simulink model "balan_model"  (R2018b)
settings: Solver=VariableStepAuto  StartTime=0.0  StopTime=15  FixedStep=0.001  MaxStep=0.01  RelTol=1e-6
undefined symbols (not defined in the file or in its folder): b, cart_d0, cart_d1, cart_d2, cart_d3, cart_d4, cart_n0, cart_n1, cart_n2, d_P_cart_den, d_P_cart_num, d_P_pend_den, d_P_pend_num, DiscIntNeverNeededParam, g, J, k, l, m, M, pend_d0, pend_d1, pend_d2, pend_d3, pend_n0, pend_n1
libraries: simulink_extras x4, simulink x3
settings Model: Creator=Ikarus  LastModifiedBy=Ikarus

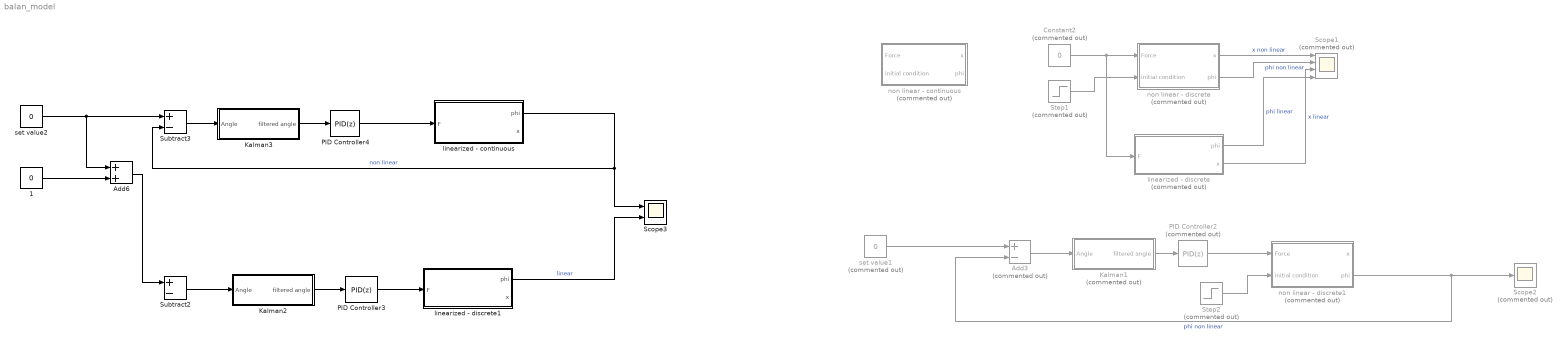
== system balan_model ==
  " 1" : Constant  Value=0  SampleTime=-1
  Add3 : Sum  Commented=on  Inputs=+-
  Add6 : Sum
  Constant2 : Constant  Commented=on  Value=0
  Kalman1 : Subsystem  Commented=on  mask{step_time=0.01}
      mask prompts: step_time "step time"
  Kalman2 : Subsystem  mask{step_time=0.01}
      mask prompts: step_time "step time"
  Kalman3 : Subsystem  mask{step_time=0.01}
      mask prompts: step_time "step time"
  PID Controller2 : simulink/Continuous/PID Controller  Commented=on  Controller=PID  Form=Parallel  TimeDomain=Discrete-time  SampleTime=-1  IntegratorMethod=Forward Euler  FilterMethod=Forward Euler  ControllerParametersSource=internal  P=1235  I=9215  D=40  UseFilter=on  N=868  TunerSelectOption=Transfer Function Based (PID Tuner App)  InitialConditionSource=internal  InitialConditionForIntegrator=0  InitialConditionForFilter=0  DifferentiatorICPrevScaledInput=0  ExternalReset=none  TrackingMode=off  Kt=1  LimitOutput=off  UpperSaturationLimit=inf  LowerSaturationLimit=-inf  LinearizeAsGain=on  AntiWindupMode=none  Kb=1  POutMin=[]  POutMax=[]  IOutMin=[]  IOutMax=[]  DOutMin=[]  DOutMax=[]  NOutMin=[]  NOutMax=[]  SumOutMin=[]  SumOutMax=[]  SaturationOutMin=[]  SaturationOutMax=[]  PParamMin=[]  PParamMax=[]  IParamMin=[]  IParamMax=[]  DParamMin=[]  DParamMax=[]  NParamMin=[]  NParamMax=[]  KbParamMin=[]  KbParamMax=[]  KtParamMin=[]  KtParamMax=[]  KbOutMin=[]  KbOutMax=[]  KtOutMin=[]  KtOutMax=[]  IntegratorOutMin=[]  IntegratorOutMax=[]  FilterOutMin=[]  FilterOutMax=[]  SumI1OutMin=[]  SumI1OutMax=[]  SumI2OutMin=[]  SumI2OutMax=[]  SumI3OutMin=[]  SumI3OutMax=[]  SumI4OutMin=[]  SumI4OutMax=[]  SumDOutMin=[]  SumDOutMax=[]  DifferentiatorOutMin=[]  DifferentiatorOutMax=[]  FilterDiffOutCoefMin=[]  FilterDiffOutCoefMax=[]  ReciprocalOutMin=[]  ReciprocalOutMax=[]  SumDenOutMin=[]  SumDenOutMax=[]  SumNumOutMin=[]  SumNumOutMax=[]  DivideOutMin=[]  DivideOutMax=[]  IntegratorContinuousStateAttributes=''  IntegratorStateMustResolveToSignalObject=off  IntegratorRTWStateStorageClass=Auto  FilterContinuousStateAttributes=''  FilterStateMustResolveToSignalObject=off  FilterRTWStateStorageClass=Auto  ParallelPVariant=InternalParameters  IdealPVariant=Disabled  IVariant=InternalParameters  DVariant=InternalParameters  IntegratorVariant=Discrete  SatVariant=Disabled  AWVariant=Passthrough  PCopyVariant=Disabled  TRVariant=Disabled  FdbkBlocksVariant=Forward  IdealPFdbkVariant=Disabled  SatFdbkVariant=Disabled  DerivativeFilterVariant=ForwardEulerFilter  NVariant=InternalParameters  NCopyVariant=Disabled  FilterICVariant=InternalICsFilter  IntegratorICVariant=InternalICs  ExternalResetVariant=Disabled  TRSumVariant=Passthrough  SumFdbkVariant=Disabled  SumVariant=Sum_PID
  PID Controller3 : simulink/Continuous/PID Controller  Controller=PID  Form=Parallel  TimeDomain=Discrete-time  SampleTime=-1  IntegratorMethod=Forward Euler  FilterMethod=Forward Euler  ControllerParametersSource=internal  P=789.794814229085  I=503.452349337569  D=303.317596444162  UseFilter=on  N=74.1133672012099  TunerSelectOption=Transfer Function Based (PID Tuner App)  InitialConditionSource=internal  InitialConditionForIntegrator=0  InitialConditionForFilter=0  DifferentiatorICPrevScaledInput=0  ExternalReset=none  TrackingMode=off  Kt=1  LimitOutput=off  UpperSaturationLimit=inf  LowerSaturationLimit=-inf  LinearizeAsGain=on  AntiWindupMode=none  Kb=1  POutMin=[]  POutMax=[]  IOutMin=[]  IOutMax=[]  DOutMin=[]  DOutMax=[]  NOutMin=[]  NOutMax=[]  SumOutMin=[]  SumOutMax=[]  SaturationOutMin=[]  SaturationOutMax=[]  PParamMin=[]  PParamMax=[]  IParamMin=[]  IParamMax=[]  DParamMin=[]  DParamMax=[]  NParamMin=[]  NParamMax=[]  KbParamMin=[]  KbParamMax=[]  KtParamMin=[]  KtParamMax=[]  KbOutMin=[]  KbOutMax=[]  KtOutMin=[]  KtOutMax=[]  IntegratorOutMin=[]  IntegratorOutMax=[]  FilterOutMin=[]  FilterOutMax=[]  SumI1OutMin=[]  SumI1OutMax=[]  SumI2OutMin=[]  SumI2OutMax=[]  SumI3OutMin=[]  SumI3OutMax=[]  SumI4OutMin=[]  SumI4OutMax=[]  SumDOutMin=[]  SumDOutMax=[]  DifferentiatorOutMin=[]  DifferentiatorOutMax=[]  FilterDiffOutCoefMin=[]  FilterDiffOutCoefMax=[]  ReciprocalOutMin=[]  ReciprocalOutMax=[]  SumDenOutMin=[]  SumDenOutMax=[]  SumNumOutMin=[]  SumNumOutMax=[]  DivideOutMin=[]  DivideOutMax=[]  IntegratorContinuousStateAttributes=''  IntegratorStateMustResolveToSignalObject=off  IntegratorRTWStateStorageClass=Auto  FilterContinuousStateAttributes=''  FilterStateMustResolveToSignalObject=off  FilterRTWStateStorageClass=Auto  ParallelPVariant=InternalParameters  IdealPVariant=Disabled  IVariant=InternalParameters  DVariant=InternalParameters  IntegratorVariant=Discrete  SatVariant=Disabled  AWVariant=Passthrough  PCopyVariant=Disabled  TRVariant=Disabled  FdbkBlocksVariant=Forward  IdealPFdbkVariant=Disabled  SatFdbkVariant=Disabled  DerivativeFilterVariant=ForwardEulerFilter  NVariant=InternalParameters  NCopyVariant=Disabled  FilterICVariant=InternalICsFilter  IntegratorICVariant=InternalICs  ExternalResetVariant=Disabled  TRSumVariant=Passthrough  SumFdbkVariant=Disabled  SumVariant=Sum_PID
  PID Controller4 : simulink/Continuous/PID Controller  Controller=PID  Form=Parallel  TimeDomain=Discrete-time  SampleTime=-1  IntegratorMethod=Forward Euler  FilterMethod=Forward Euler  ControllerParametersSource=internal  P=94.3174432822609  I=179.101520876593  D=7.29108455594587  UseFilter=on  N=1162.58764416015  TunerSelectOption=Transfer Function Based (PID Tuner App)  InitialConditionSource=internal  InitialConditionForIntegrator=0  InitialConditionForFilter=0  DifferentiatorICPrevScaledInput=0  ExternalReset=none  TrackingMode=off  Kt=1  LimitOutput=off  UpperSaturationLimit=inf  LowerSaturationLimit=-inf  LinearizeAsGain=on  AntiWindupMode=none  Kb=1  POutMin=[]  POutMax=[]  IOutMin=[]  IOutMax=[]  DOutMin=[]  DOutMax=[]  NOutMin=[]  NOutMax=[]  SumOutMin=[]  SumOutMax=[]  SaturationOutMin=[]  SaturationOutMax=[]  PParamMin=[]  PParamMax=[]  IParamMin=[]  IParamMax=[]  DParamMin=[]  DParamMax=[]  NParamMin=[]  NParamMax=[]  KbParamMin=[]  KbParamMax=[]  KtParamMin=[]  KtParamMax=[]  KbOutMin=[]  KbOutMax=[]  KtOutMin=[]  KtOutMax=[]  IntegratorOutMin=[]  IntegratorOutMax=[]  FilterOutMin=[]  FilterOutMax=[]  SumI1OutMin=[]  SumI1OutMax=[]  SumI2OutMin=[]  SumI2OutMax=[]  SumI3OutMin=[]  SumI3OutMax=[]  SumI4OutMin=[]  SumI4OutMax=[]  SumDOutMin=[]  SumDOutMax=[]  DifferentiatorOutMin=[]  DifferentiatorOutMax=[]  FilterDiffOutCoefMin=[]  FilterDiffOutCoefMax=[]  ReciprocalOutMin=[]  ReciprocalOutMax=[]  SumDenOutMin=[]  SumDenOutMax=[]  SumNumOutMin=[]  SumNumOutMax=[]  DivideOutMin=[]  DivideOutMax=[]  IntegratorContinuousStateAttributes=''  IntegratorStateMustResolveToSignalObject=off  IntegratorRTWStateStorageClass=Auto  FilterContinuousStateAttributes=''  FilterStateMustResolveToSignalObject=off  FilterRTWStateStorageClass=Auto  ParallelPVariant=InternalParameters  IdealPVariant=Disabled  IVariant=InternalParameters  DVariant=InternalParameters  IntegratorVariant=Discrete  SatVariant=Disabled  AWVariant=Passthrough  PCopyVariant=Disabled  TRVariant=Disabled  FdbkBlocksVariant=Forward  IdealPFdbkVariant=Disabled  SatFdbkVariant=Disabled  DerivativeFilterVariant=ForwardEulerFilter  NVariant=InternalParameters  NCopyVariant=Disabled  FilterICVariant=InternalICsFilter  IntegratorICVariant=InternalICs  ExternalResetVariant=Disabled  TRSumVariant=Passthrough  SumFdbkVariant=Disabled  SumVariant=Sum_PID
  Scope1 : Scope  Commented=on  NumInputPorts=4
  Scope2 : Scope  Commented=on
  Scope3 : Scope  NumInputPorts=2
  Step1 : Step  Commented=on  Before=10*pi/180  After=0  SampleTime=0
  Step2 : Step  Commented=on  Before=10*pi/180  After=0  SampleTime=0
  Subtract2 : Sum  Inputs=+-
  Subtract3 : Sum  Inputs=+-
  linearized - continuous : Subsystem
  linearized - discrete : Subsystem  Commented=on
  linearized - discrete1 : Subsystem
  non linear - continuous : Subsystem  Commented=on
  non linear - discrete : Subsystem  Commented=on
  non linear - discrete1 : Subsystem  Commented=on
  set value1 : Constant  Commented=on  Value=0
  set value2 : Constant  Value=0  SampleTime=-1
  wires:
  non linear - discrete/1(x) -> Scope1/1  "x non linear"
  non linear - discrete/2(phi) -> Scope1/2  "phi non linear"
  Constant2/1 -> linearized - discrete/1(F), non linear - discrete/1("Force ")
  linearized - discrete/1(phi) -> Scope1/4  "phi linear"
  linearized - discrete/2(x) -> Scope1/3  "x linear"
  Step1/1 -> non linear - discrete/2("initial condition ")
  PID Controller2/1 -> non linear - discrete1/1("Force ")
  Step2/1 -> non linear - discrete1/2("initial condition ")
  non linear - discrete1/2(phi) -> Scope2/1, Add3/2  "phi non linear"
  set value1/1 -> Add3/1
  Kalman1/1(filtered angle) -> PID Controller2/1
  Add3/1 -> Kalman1/1("Angle ")
  Add6/1 -> Subtract2/1
  linearized - continuous/1(phi) -> Subtract3/2, Scope3/1  "non linear"
  set value2/1 -> Subtract3/1, Add6/1
  " 1"/1 -> Add6/2
  Kalman3/1(filtered angle) -> PID Controller4/1
  Subtract3/1 -> Kalman3/1("Angle ")
  PID Controller4/1 -> linearized - continuous/1(F)
  Subtract2/1 -> Kalman2/1("Angle ")
  PID Controller3/1 -> linearized - discrete1/1(F)
  linearized - discrete1/1(phi) -> Scope3/2  "linear"
  Kalman2/1(filtered angle) -> PID Controller3/1

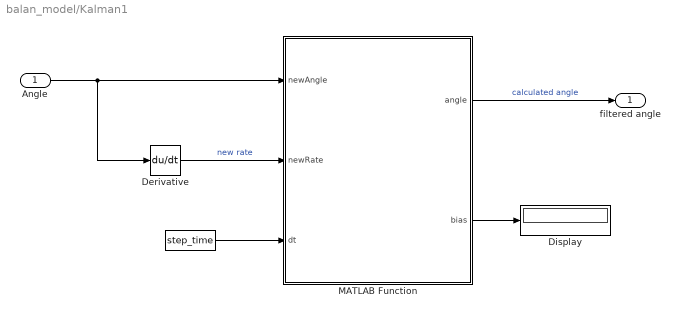
== system balan_model/Kalman1 ==
  "Angle " : Inport
  "  " : Constant  Value=step_time
  Derivative : Derivative
  Display : Display
  MATLAB Function : MATLAB Function  TreatAsAtomicUnit=on
  filtered angle : Outport
  wires:
  "  "/1 -> MATLAB Function/3(dt)
  Derivative/1 -> MATLAB Function/2(newRate)  "new rate"
  MATLAB Function/1(angle) -> filtered angle/1  "calculated angle"
  "Angle "/1 -> Derivative/1, MATLAB Function/1(newAngle)
  MATLAB Function/2(bias) -> Display/1

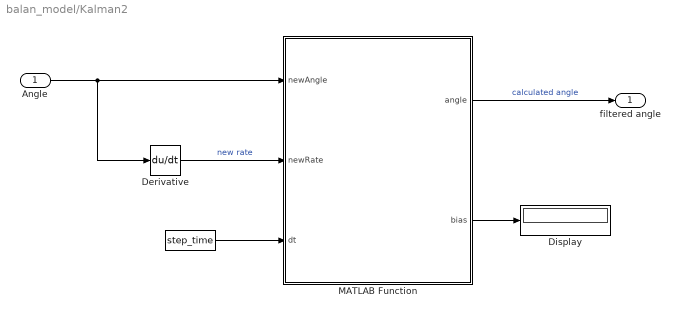
== system balan_model/Kalman2 ==
  "Angle " : Inport
  "  " : Constant  Value=step_time  SampleTime=-1
  Derivative : Derivative  CoefficientInTFapproximation=-1
  Display : Display
  MATLAB Function : MATLAB Function  TreatAsAtomicUnit=on
  filtered angle : Outport
  wires:
  MATLAB Function/2(bias) -> Display/1
  "Angle "/1 -> MATLAB Function/1(newAngle), Derivative/1
  MATLAB Function/1(angle) -> filtered angle/1  "calculated angle"
  Derivative/1 -> MATLAB Function/2(newRate)  "new rate"
  "  "/1 -> MATLAB Function/3(dt)

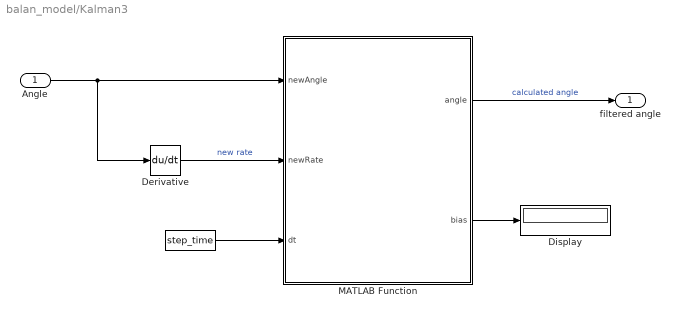
== system balan_model/Kalman3 ==
  "Angle " : Inport
  "  " : Constant  Value=step_time
  Derivative : Derivative
  Display : Display
  MATLAB Function : MATLAB Function  TreatAsAtomicUnit=on
  filtered angle : Outport
  wires:
  "  "/1 -> MATLAB Function/3(dt)
  Derivative/1 -> MATLAB Function/2(newRate)  "new rate"
  MATLAB Function/1(angle) -> filtered angle/1  "calculated angle"
  "Angle "/1 -> Derivative/1, MATLAB Function/1(newAngle)
  MATLAB Function/2(bias) -> Display/1

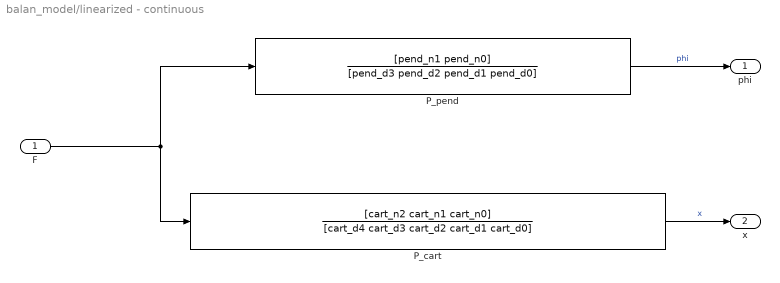
== system balan_model/linearized - continuous ==
  F : Inport
  P_cart : TransferFcn  Numerator=[cart_n2 cart_n1 cart_n0]  Denominator=[cart_d4 cart_d3 cart_d2 cart_d1 cart_d0]
  P_pend : TransferFcn  Numerator=[pend_n1 pend_n0]  Denominator=[pend_d3 pend_d2 pend_d1 pend_d0]
  phi : Outport
  x : Outport  Port=2
  wires:
  P_cart/1 -> x/1  "x"
  F/1 -> P_pend/1, P_cart/1
  P_pend/1 -> phi/1  "phi"

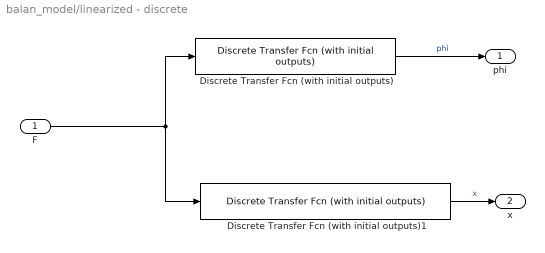
== system balan_model/linearized - discrete ==
  F : Inport
  Discrete Transfer Fcn (with initial outputs) : simulink_extras/Additional Discrete/Discrete Transfer Fcn (with initial outputs)  N=[d_P_pend_num]  D=[d_P_pend_den]  U0=0  Y0=10  TS=-1
      settings: SourceProductName=Simulink  SourceProductBaseCode=SL
  Discrete Transfer Fcn (with initial outputs)1 : simulink_extras/Additional Discrete/Discrete Transfer Fcn (with initial outputs)  N=[d_P_cart_num]  D=[d_P_cart_den]  U0=0  Y0=0  TS=-1
      settings: SourceProductName=Simulink  SourceProductBaseCode=SL
  phi : Outport
  x : Outport  Port=2
  wires:
  Discrete Transfer Fcn (with initial outputs)/1 -> phi/1  "phi"
  Discrete Transfer Fcn (with initial outputs)1/1 -> x/1  "x"
  F/1 -> Discrete Transfer Fcn (with initial outputs)1/1, Discrete Transfer Fcn (with initial outputs)/1

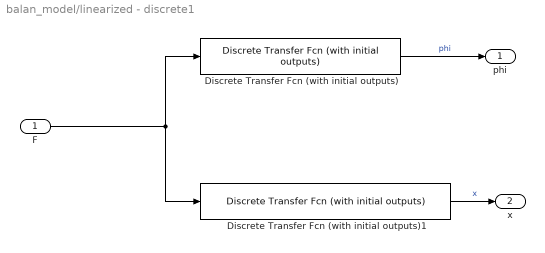
== system balan_model/linearized - discrete1 ==
  F : Inport
  Discrete Transfer Fcn (with initial outputs) : simulink_extras/Additional Discrete/Discrete Transfer Fcn (with initial outputs)  N=[d_P_pend_num]  D=[d_P_pend_den]  U0=0  Y0=10*pi/180  TS=-1
      settings: SourceProductName=Simulink  SourceProductBaseCode=SL
  Discrete Transfer Fcn (with initial outputs)1 : simulink_extras/Additional Discrete/Discrete Transfer Fcn (with initial outputs)  N=[d_P_cart_num]  D=[d_P_cart_den]  U0=0  Y0=0  TS=-1
      settings: SourceProductName=Simulink  SourceProductBaseCode=SL
  phi : Outport
  x : Outport  Port=2
  wires:
  F/1 -> Discrete Transfer Fcn (with initial outputs)/1, Discrete Transfer Fcn (with initial outputs)1/1
  Discrete Transfer Fcn (with initial outputs)1/1 -> x/1  "x"
  Discrete Transfer Fcn (with initial outputs)/1 -> phi/1  "phi"

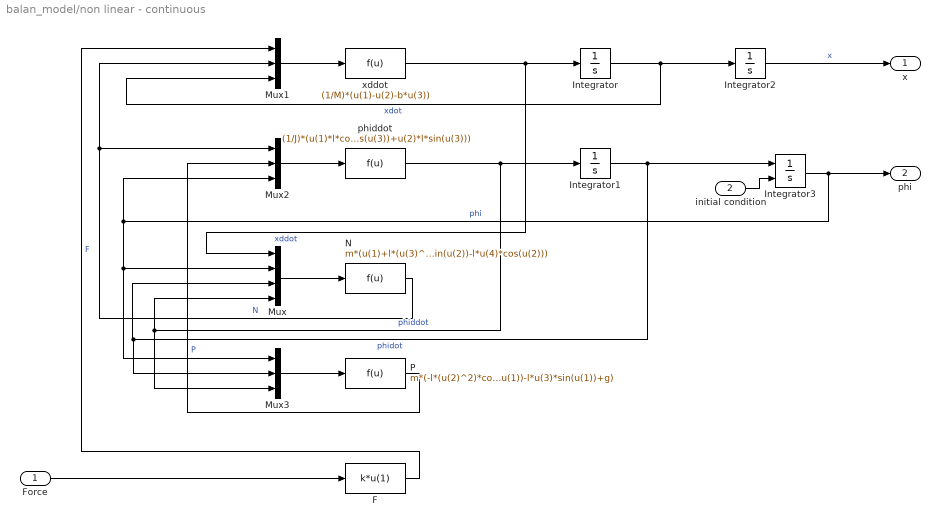
== system balan_model/non linear - continuous ==
  "Force " : Inport
  "initial condition " : Inport  Port=2
  F : Fcn  Expr=k*u(1)
  Integrator : Integrator
  Integrator1 : Integrator
  Integrator2 : Integrator
  Integrator3 : Integrator  InitialConditionSource=external  InitialCondition=pi/36
  Mux : Mux
  Mux1 : Mux  Inputs=3
  Mux2 : Mux  Inputs=3
  Mux3 : Mux  Inputs=3
  N : Fcn  Expr=m*(u(1)+l*(u(3)^2)*sin(u(2))-l*u(4)*cos(u(2)))
  P : Fcn  Expr=m*(-l*(u(2)^2)*cos(u(1))-l*u(3)*sin(u(1))+g)
  phiddot : Fcn  Expr=(1/J)*(u(1)*l*cos(u(3))+u(2)*l*sin(u(3)))
  xddot : Fcn  Expr=(1/M)*(u(1)-u(2)-b*u(3))
  x : Outport
  phi : Outport  Port=2
  wires:
  Mux2/1 -> phiddot/1
  Integrator1/1 -> Integrator3/1, Mux3/2, Mux/3  "phidot"
  "Force "/1 -> F/1
  Integrator3/1 -> phi/1, Mux2/3, Mux3/1, Mux/2  "phi"
  Integrator/1 -> Integrator2/1, Mux1/3  "xdot"
  Mux/1 -> N/1
  F/1 -> Mux1/1  "F"
  xddot/1 -> Mux/1, Integrator/1  "xddot"
  P/1 -> Mux2/2  "P"
  Integrator2/1 -> x/1  "x"
  N/1 -> Mux1/2, Mux2/1  "N"
  phiddot/1 -> Mux3/3, Mux/4, Integrator1/1  "phiddot"
  Mux1/1 -> xddot/1
  Mux3/1 -> P/1
  "initial condition "/1 -> Integrator3/2

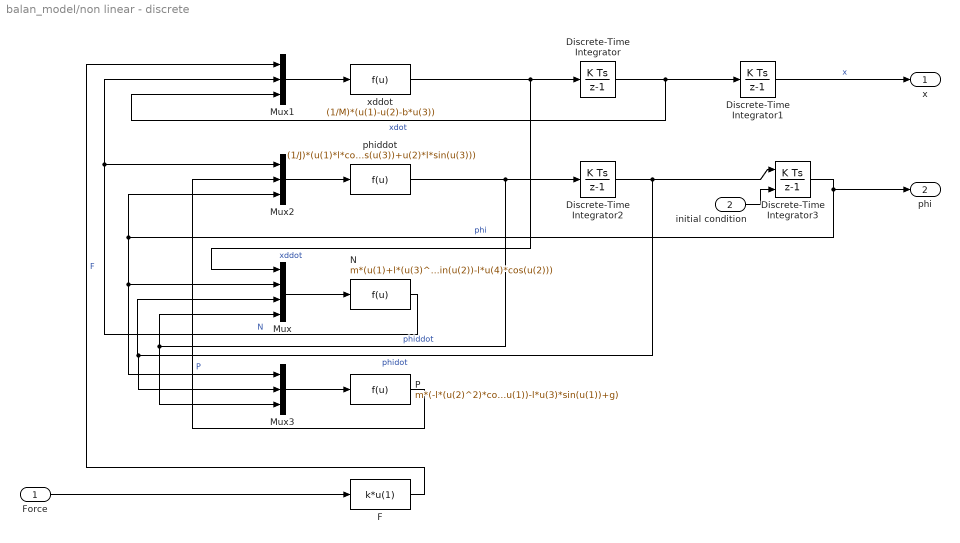
== system balan_model/non linear - discrete ==
  "Force " : Inport
  "initial condition " : Inport  Port=2
  Discrete-Time Integrator : DiscreteIntegrator  SampleTime=-1  ICPrevOutput=DiscIntNeverNeededParam  ICPrevScaledInput=DiscIntNeverNeededParam
  Discrete-Time Integrator1 : DiscreteIntegrator  SampleTime=-1  ICPrevOutput=DiscIntNeverNeededParam  ICPrevScaledInput=DiscIntNeverNeededParam
  Discrete-Time Integrator2 : DiscreteIntegrator  SampleTime=-1  ICPrevOutput=DiscIntNeverNeededParam  ICPrevScaledInput=DiscIntNeverNeededParam
  Discrete-Time Integrator3 : DiscreteIntegrator  InitialConditionSource=external  SampleTime=-1  ICPrevOutput=DiscIntNeverNeededParam  ICPrevScaledInput=DiscIntNeverNeededParam
  F : Fcn  Expr=k*u(1)
  Mux : Mux
  Mux1 : Mux  Inputs=3
  Mux2 : Mux  Inputs=3
  Mux3 : Mux  Inputs=3
  N : Fcn  Expr=m*(u(1)+l*(u(3)^2)*sin(u(2))-l*u(4)*cos(u(2)))
  P : Fcn  Expr=m*(-l*(u(2)^2)*cos(u(1))-l*u(3)*sin(u(1))+g)
  phiddot : Fcn  Expr=(1/J)*(u(1)*l*cos(u(3))+u(2)*l*sin(u(3)))
  xddot : Fcn  Expr=(1/M)*(u(1)-u(2)-b*u(3))
  x : Outport
  phi : Outport  Port=2
  wires:
  phiddot/1 -> Discrete-Time Integrator2/1, Mux3/3, Mux/4  "phiddot"
  N/1 -> Mux1/2, Mux2/1  "N"
  Discrete-Time Integrator3/1 -> phi/1, Mux2/3, Mux3/1, Mux/2  "phi"
  Discrete-Time Integrator/1 -> Discrete-Time Integrator1/1, Mux1/3  "xdot"
  Discrete-Time Integrator2/1 -> Discrete-Time Integrator3/1, Mux3/2, Mux/3  "phidot"
  xddot/1 -> Discrete-Time Integrator/1, Mux/1  "xddot"
  Mux1/1 -> xddot/1
  Mux2/1 -> phiddot/1
  "Force "/1 -> F/1
  P/1 -> Mux2/2  "P"
  Mux/1 -> N/1
  Mux3/1 -> P/1
  F/1 -> Mux1/1  "F"
  "initial condition "/1 -> Discrete-Time Integrator3/2
  Discrete-Time Integrator1/1 -> x/1  "x"

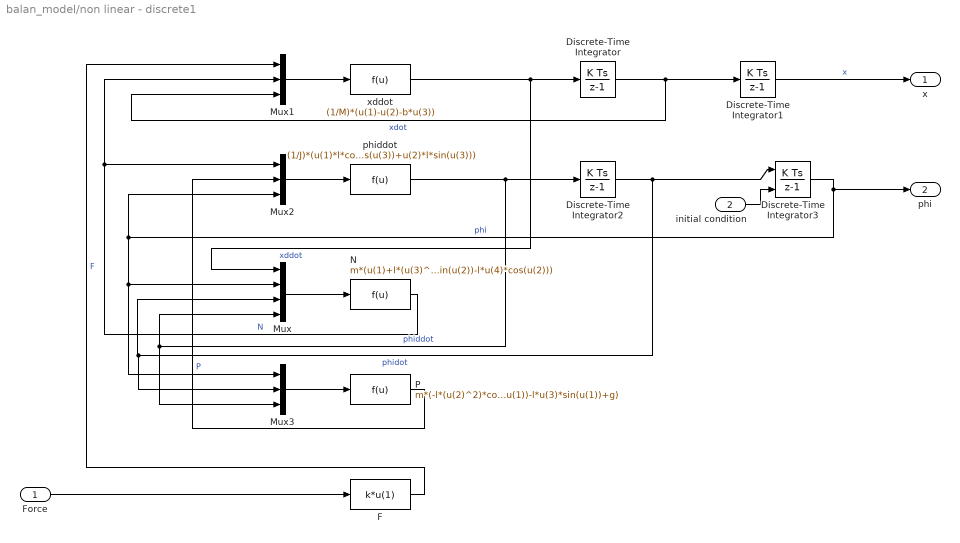
== system balan_model/non linear - discrete1 ==
  "Force " : Inport
  "initial condition " : Inport  Port=2
  Discrete-Time Integrator : DiscreteIntegrator  SampleTime=-1  ICPrevOutput=DiscIntNeverNeededParam  ICPrevScaledInput=DiscIntNeverNeededParam
  Discrete-Time Integrator1 : DiscreteIntegrator  SampleTime=-1  ICPrevOutput=DiscIntNeverNeededParam  ICPrevScaledInput=DiscIntNeverNeededParam
  Discrete-Time Integrator2 : DiscreteIntegrator  SampleTime=-1  ICPrevOutput=DiscIntNeverNeededParam  ICPrevScaledInput=DiscIntNeverNeededParam
  Discrete-Time Integrator3 : DiscreteIntegrator  InitialConditionSource=external  SampleTime=-1  ICPrevOutput=DiscIntNeverNeededParam  ICPrevScaledInput=DiscIntNeverNeededParam
  F : Fcn  Expr=k*u(1)
  Mux : Mux
  Mux1 : Mux  Inputs=3
  Mux2 : Mux  Inputs=3
  Mux3 : Mux  Inputs=3
  N : Fcn  Expr=m*(u(1)+l*(u(3)^2)*sin(u(2))-l*u(4)*cos(u(2)))
  P : Fcn  Expr=m*(-l*(u(2)^2)*cos(u(1))-l*u(3)*sin(u(1))+g)
  phiddot : Fcn  Expr=(1/J)*(u(1)*l*cos(u(3))+u(2)*l*sin(u(3)))
  xddot : Fcn  Expr=(1/M)*(u(1)-u(2)-b*u(3))
  x : Outport
  phi : Outport  Port=2
  wires:
  Discrete-Time Integrator1/1 -> x/1  "x"
  "initial condition "/1 -> Discrete-Time Integrator3/2
  F/1 -> Mux1/1  "F"
  Mux3/1 -> P/1
  Mux/1 -> N/1
  P/1 -> Mux2/2  "P"
  "Force "/1 -> F/1
  Mux2/1 -> phiddot/1
  Mux1/1 -> xddot/1
  xddot/1 -> Mux/1, Discrete-Time Integrator/1  "xddot"
  Discrete-Time Integrator2/1 -> Mux/3, Mux3/2, Discrete-Time Integrator3/1  "phidot"
  Discrete-Time Integrator/1 -> Mux1/3, Discrete-Time Integrator1/1  "xdot"
  Discrete-Time Integrator3/1 -> Mux/2, Mux3/1, Mux2/3, phi/1  "phi"
  N/1 -> Mux2/1, Mux1/2  "N"
  phiddot/1 -> Mux/4, Mux3/3, Discrete-Time Integrator2/1  "phiddot"

== matlab function balan_model/Kalman1/MATLAB Function ==
  settings: updateMethod=DISCRETE
  data: newAngle input; angle output; newRate input; dt input; bias output
function [angle,bias] = KalmanFil_Balanbot(newAngle,newRate,dt)
        % This script was adapted for its implementation in Simulink by R. Estrada (FH JOANNEUM 2017)
        % Based on KasBot V2  -  Kalman filter module - http:%www.x-firm.com/?page_id=145
        % Modified by Kristian Lauszus
        % More information: http:%blog.tkjelectronics.dk/2012/09/a-practical-approach-to-kalman-filter-and-how-to-implement-it

        % Discrete Kalman filter time update equations - Time Update ("Predict")
        % Update xhat - Project the state ahead
        
        coder.extrinsic('exist');
        
        % Declaration of persistent in memory variables (similar to declare global
        % variables)
   
        persistent init0 P K x;        
        
        % Initialization of typical sensor and noise variances 
        Q_angle = 0.001;
        Q_bias = 0.003; 
        R_measure = 0.03;
        
        % Declaration/initialization of main static matrices and vectors
        F = [1      -dt; 0      1];     % Transition matrix
        Q = [Q_angle  0; 0 Q_bias];     % Process noise covariance matrix  
        B = [dt ; 0];                   % Control-input model
        H = [1    0];                   % Observation model
        
        % SETUP: Executed only the first time      
        if isempty(init0)
            init0=0;
             % Declaration/initialization of main dynamic matrix and vectors
            P     = [0 0;0 0];  % Error covariance matrix
            K     = [0;0];      % Kalman gain vector
            x     = [0;0];      % State vector
        end

        % LOOP: Implementation of Kalman filter algorithm
        
        % Step 1 */          
        % Calculate prior state vector
        x = F * x + B * newRate;        

        % Step 2 */ 
        % Update estimation error covariance - Project the error covariance ahead               
         P = F * P * F' + Q * dt;  
                   
        % Step 3 */
        % Update estimate with measurement zk (newAngle)     
        y = newAngle - H * x;
        
        % Step 4 */
        % Discrete Kalman filter measurement update equations - Measurement Update ("Correct")              
        S = H * P * H' + R_measure;
        
        % Step 5 */
        % Compute the Kalman gain  
        K = P * H' / S;

        % Step 6 */
        % Update state vector
        x = x + K * y;
        
        % Step 7 */
        % Calculate estimation error covariance - Update the error covariance
        P = (eye(2) - K * H) * P;

        % RETURN: Update the function outputs
        angle = x(1);
        bias  = x(2);

== matlab function balan_model/Kalman3/MATLAB Function ==
  settings: updateMethod=DISCRETE
  data: newAngle input; angle output; newRate input; dt input; bias output
function [angle,bias] = KalmanFil_Balanbot(newAngle,newRate,dt)
        % This script was adapted for its implementation in Simulink by R. Estrada (FH JOANNEUM 2017)
        % Based on KasBot V2  -  Kalman filter module - http:%www.x-firm.com/?page_id=145
        % Modified by Kristian Lauszus
        % More information: http:%blog.tkjelectronics.dk/2012/09/a-practical-approach-to-kalman-filter-and-how-to-implement-it

        % Discrete Kalman filter time update equations - Time Update ("Predict")
        % Update xhat - Project the state ahead
        
        coder.extrinsic('exist');
        
        % Declaration of persistent in memory variables (similar to declare global
        % variables)
   
        persistent init0 P K x;        
        
        % Initialization of typical sensor and noise variances 
        Q_angle = 0.001;
        Q_bias = 0.003; 
        R_measure = 0.03;
        
        % Declaration/initialization of main static matrices and vectors
        F = [1      -dt; 0      1];     % Transition matrix
        Q = [Q_angle  0; 0 Q_bias];     % Process noise covariance matrix  
        B = [dt ; 0];                   % Control-input model
        H = [1    0];                   % Observation model
        
        % SETUP: Executed only the first time      
        if isempty(init0)
            init0=0;
             % Declaration/initialization of main dynamic matrix and vectors
            P     = [0 0;0 0];  % Error covariance matrix
            K     = [0;0];      % Kalman gain vector
            x     = [0;0];      % State vector
        end

        % LOOP: Implementation of Kalman filter algorithm
        
        % Step 1 */          
        % Calculate prior state vector
        x = F * x + B * newRate;        

        % Step 2 */ 
        % Update estimation error covariance - Project the error covariance ahead               
         P = F * P * F' + Q * dt;  
                   
        % Step 3 */
        % Update estimate with measurement zk (newAngle)     
        y = newAngle - H * x;
        
        % Step 4 */
        % Discrete Kalman filter measurement update equations - Measurement Update ("Correct")              
        S = H * P * H' + R_measure;
        
        % Step 5 */
        % Compute the Kalman gain  
        K = P * H' / S;

        % Step 6 */
        % Update state vector
        x = x + K * y;
        
        % Step 7 */
        % Calculate estimation error covariance - Update the error covariance
        P = (eye(2) - K * H) * P;

        % RETURN: Update the function outputs
        angle = x(1);
        bias  = x(2);

== matlab function balan_model/Kalman2/MATLAB Function ==
  settings: updateMethod=DISCRETE
  data: newAngle input; angle output; newRate input; dt input; bias output
function [angle,bias] = KalmanFil_Balanbot(newAngle,newRate,dt)
        % This script was adapted for its implementation in Simulink by R. Estrada (FH JOANNEUM 2017)
        % Based on KasBot V2  -  Kalman filter module - http:%www.x-firm.com/?page_id=145
        % Modified by Kristian Lauszus
        % More information: http:%blog.tkjelectronics.dk/2012/09/a-practical-approach-to-kalman-filter-and-how-to-implement-it

        % Discrete Kalman filter time update equations - Time Update ("Predict")
        % Update xhat - Project the state ahead
        
        coder.extrinsic('exist');
        
        % Declaration of persistent in memory variables (similar to declare global
        % variables)
   
        persistent init0 P K x;        
        
        % Initialization of typical sensor and noise variances 
        Q_angle = 0.001;
        Q_bias = 0.003; 
        R_measure = 0.03;
        
        % Declaration/initialization of main static matrices and vectors
        F = [1      -dt; 0      1];     % Transition matrix
        Q = [Q_angle  0; 0 Q_bias];     % Process noise covariance matrix  
        B = [dt ; 0];                   % Control-input model
        H = [1    0];                   % Observation model
        
        % SETUP: Executed only the first time      
        if isempty(init0)
            init0=0;
             % Declaration/initialization of main dynamic matrix and vectors
            P     = [0 0;0 0];  % Error covariance matrix
            K     = [0;0];      % Kalman gain vector
            x     = [0;0];      % State vector
        end

        % LOOP: Implementation of Kalman filter algorithm
        
        % Step 1 */          
        % Calculate prior state vector
        x = F * x + B * newRate;        

        % Step 2 */ 
        % Update estimation error covariance - Project the error covariance ahead               
         P = F * P * F' + Q * dt;  
                   
        % Step 3 */
        % Update estimate with measurement zk (newAngle)     
        y = newAngle - H * x;
        
        % Step 4 */
        % Discrete Kalman filter measurement update equations - Measurement Update ("Correct")              
        S = H * P * H' + R_measure;
        
        % Step 5 */
        % Compute the Kalman gain  
        K = P * H' / S;

        % Step 6 */
        % Update state vector
        x = x + K * y;
        
        % Step 7 */
        % Calculate estimation error covariance - Update the error covariance
        P = (eye(2) - K * H) * P;

        % RETURN: Update the function outputs
        angle = x(1);
        bias  = x(2);
